simulink model "ModelSimulink"  (R2020a)
settings: Solver=VariableStepAuto  StartTime=0.0  StopTime=20  RelTol=1e-3
libraries: robotlib x50
settings Model: Creator=Ishmael  LastModifiedBy=Ishmael

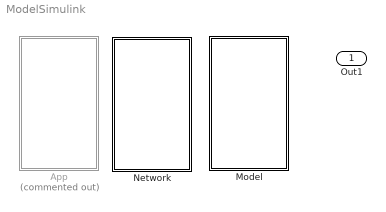
== system ModelSimulink ==
  App : Subsystem  Commented=on
  Model : Subsystem
  Network : Subsystem
  Out1 : Outport

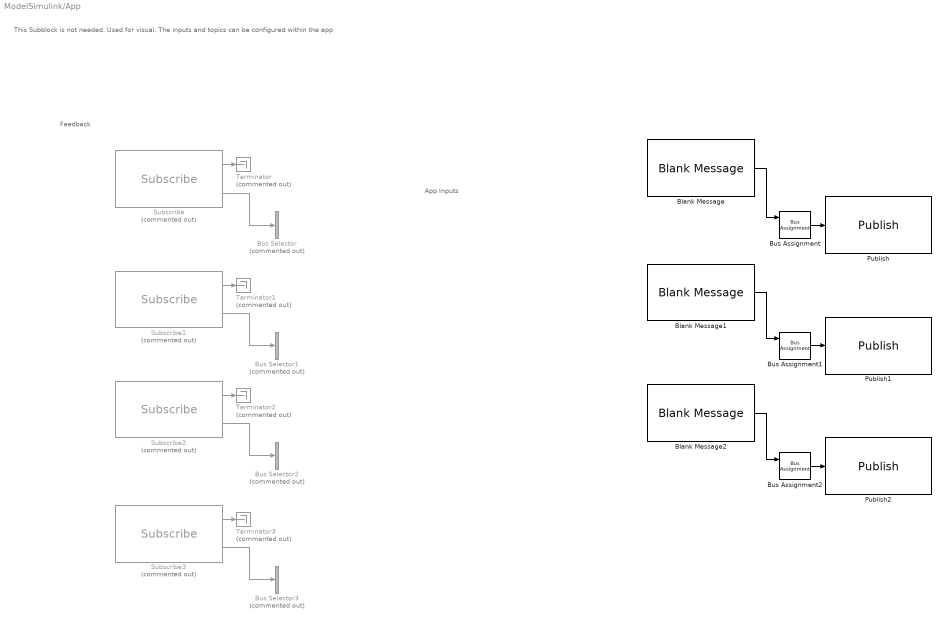
== system ModelSimulink/App ==
  note: This Subblock is not needed. Used for visual. The inputs and topics can be configured within the app
  note: App Inputs
  note: Feedback
  Blank Message : robotlib/Blank Message  messageClass=Message  entityType=geometry_msgs/Twist  messageType=geometry_msgs/Twist  SampleTime=inf
  Blank Message1 : robotlib/Blank Message  messageClass=Message  entityType=geometry_msgs/Twist  messageType=geometry_msgs/Twist  SampleTime=inf
  Blank Message2 : robotlib/Blank Message  messageClass=Message  entityType=geometry_msgs/Twist  messageType=geometry_msgs/Twist  SampleTime=inf
  Bus Assignment : BusAssignment  AssignedSignals=Linear.X
  Bus Assignment1 : BusAssignment  AssignedSignals=Linear.X
  Bus Assignment2 : BusAssignment  AssignedSignals=Linear.X
  Bus Selector{,1..3} (4 alike) : BusSelector  Commented=on  OutputSignals=Linear.X
  Publish : robotlib/Publish  topicSource=Select from ROS network  topic=/App/PedalPositionCommand  messageType=geometry_msgs/Twist  messageQueueLength=1
  Publish1 : robotlib/Publish  topicSource=Select from ROS network  topic=/App/SteeringPositionCommand  messageType=geometry_msgs/Twist  messageQueueLength=1
  Publish2 : robotlib/Publish  topicSource=Select from ROS network  topic=/App/SteeringPositionCommand  messageType=geometry_msgs/Twist  messageQueueLength=1
  Subscribe : robotlib/Subscribe  Commented=on  topicSource=Select from ROS network  topic=/App/CurrentPedalPosition  messageType=geometry_msgs/Twist  sampleTime=-1  messageQueueLength=1
  Subscribe1 : robotlib/Subscribe  Commented=on  topicSource=Select from ROS network  topic=/App/CurrentSteeringPosition  messageType=geometry_msgs/Twist  sampleTime=-1  messageQueueLength=1
  Subscribe2 : robotlib/Subscribe  Commented=on  topicSource=Select from ROS network  topic=/App/CurrentBreakingPosition  messageType=geometry_msgs/Twist  sampleTime=-1  messageQueueLength=1
  Subscribe3 : robotlib/Subscribe  Commented=on  topicSource=Select from ROS network  topic=/Model/Camera  messageType=geometry_msgs/Twist  sampleTime=-1  messageQueueLength=1
  Terminator{,1..3} (4 alike) : Terminator  Commented=on
  wires:
  Bus Assignment/1 -> Publish/1
  Blank Message/1 -> Bus Assignment/1
  ? -> Bus Assignment/2
  ? -> Bus Assignment1/2
  Blank Message1/1 -> Bus Assignment1/1
  Bus Assignment1/1 -> Publish1/1
  Bus Assignment2/1 -> Publish2/1
  Blank Message2/1 -> Bus Assignment2/1
  ? -> Bus Assignment2/2
  Subscribe/1 -> Terminator/1
  Subscribe/2 -> Bus Selector/1
  Subscribe1/2 -> Bus Selector1/1
  Subscribe1/1 -> Terminator1/1
  Subscribe2/1 -> Terminator2/1
  Subscribe2/2 -> Bus Selector2/1
  Subscribe3/2 -> Bus Selector3/1
  Subscribe3/1 -> Terminator3/1

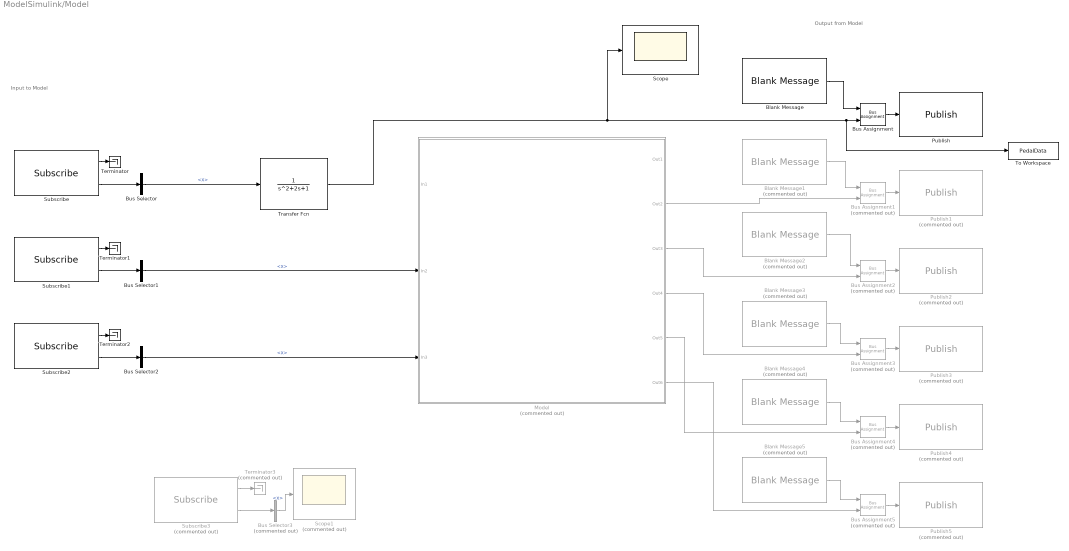
== system ModelSimulink/Model ==
  note: Input to Model
  note: Output from Model
  Blank Message : robotlib/Blank Message  messageClass=Message  entityType=geometry_msgs/Twist  messageType=geometry_msgs/Twist  SampleTime=inf
  Blank Message{1..5} (5 alike) : robotlib/Blank Message  Commented=on  messageClass=Message  entityType=geometry_msgs/Twist  messageType=geometry_msgs/Twist  SampleTime=inf
  Bus Assignment : BusAssignment  AssignedSignals=Linear.X
  Bus Assignment{1..5} (5 alike) : BusAssignment  Commented=on  AssignedSignals=Linear.X
  Bus Selector : BusSelector  OutputSignals=Linear.X
  Bus Selector1 : BusSelector  OutputSignals=Linear.X
  Bus Selector2 : BusSelector  OutputSignals=Linear.X
  Bus Selector3 : BusSelector  Commented=on  OutputSignals=Linear.X
  Model : Subsystem  Commented=on
  Publish : robotlib/Publish  topicSource=Select from ROS network  topic=/Model/PedalPositionReturn  messageType=geometry_msgs/Twist  messageQueueLength=1
  Publish1 : robotlib/Publish  Commented=on  topicSource=Select from ROS network  topic=/Model/SteeringPositionReturn  messageType=geometry_msgs/Twist  messageQueueLength=1
  Publish2 : robotlib/Publish  Commented=on  topicSource=Select from ROS network  topic=/Model/BreakingPositionReturn  messageType=geometry_msgs/Twist  messageQueueLength=1
  Publish3 : robotlib/Publish  Commented=on  topicSource=Select from ROS network  topic=/Model/Acceleration  messageType=geometry_msgs/Twist  messageQueueLength=1
  Publish4 : robotlib/Publish  Commented=on  topicSource=Select from ROS network  topic=/Model/TireAngle  messageType=geometry_msgs/Twist  messageQueueLength=1
  Publish5 : robotlib/Publish  Commented=on  topicSource=Select from ROS network  topic=/Model/Camera  messageType=geometry_msgs/Twist  messageQueueLength=1
  Scope : Scope
  Scope1 : Scope  Commented=on
  Subscribe : robotlib/Subscribe  topicSource=Select from ROS network  topic=/PedalPositionSend2m  messageType=geometry_msgs/Twist  sampleTime=-1  messageQueueLength=1
  Subscribe1 : robotlib/Subscribe  topicSource=Select from ROS network  topic=/SteeringPositionSend2m  messageType=geometry_msgs/Twist  sampleTime=-1  messageQueueLength=1
  Subscribe2 : robotlib/Subscribe  topicSource=Select from ROS network  topic=/BreakingPositionSend2m  messageType=geometry_msgs/Twist  sampleTime=-1  messageQueueLength=1
  Subscribe3 : robotlib/Subscribe  Commented=on  topicSource=Select from ROS network  topic=/Model/PedalPositionReturn  messageType=geometry_msgs/Twist  sampleTime=-1  messageQueueLength=1
  Terminator : Terminator
  Terminator1 : Terminator
  Terminator2 : Terminator
  Terminator3 : Terminator  Commented=on
  To Workspace : ToWorkspace  VariableName=PedalData  SaveFormat=Timeseries  SampleTime=-1
  Transfer Fcn : TransferFcn
  wires:
  Subscribe/1 -> Terminator/1
  Subscribe/2 -> Bus Selector/1
  Subscribe1/2 -> Bus Selector1/1
  Subscribe1/1 -> Terminator1/1
  Subscribe2/1 -> Terminator2/1
  Subscribe2/2 -> Bus Selector2/1
  Bus Selector2/1 -> Model/3(In3)  "<X>"
  Bus Selector/1 -> Transfer Fcn/1  "<X>"
  Bus Selector1/1 -> Model/2(In2)  "<X>"
  Bus Assignment/1 -> Publish/1
  Blank Message/1 -> Bus Assignment/1
  Model/2(Out2) -> Bus Assignment1/2
  Blank Message1/1 -> Bus Assignment1/1
  Bus Assignment1/1 -> Publish1/1
  Bus Assignment2/1 -> Publish2/1
  Blank Message2/1 -> Bus Assignment2/1
  Model/3(Out3) -> Bus Assignment2/2
  Model/4(Out4) -> Bus Assignment3/2
  Blank Message3/1 -> Bus Assignment3/1
  Bus Assignment3/1 -> Publish3/1
  Bus Assignment4/1 -> Publish4/1
  Blank Message4/1 -> Bus Assignment4/1
  Model/5(Out5) -> Bus Assignment4/2
  Model/6(Out6) -> Bus Assignment5/2
  Blank Message5/1 -> Bus Assignment5/1
  Bus Assignment5/1 -> Publish5/1
  Transfer Fcn/1 -> Scope/1, To Workspace/1, Bus Assignment/2
  Subscribe3/1 -> Terminator3/1
  Subscribe3/2 -> Bus Selector3/1
  Bus Selector3/1 -> Scope1/1  "<X>"

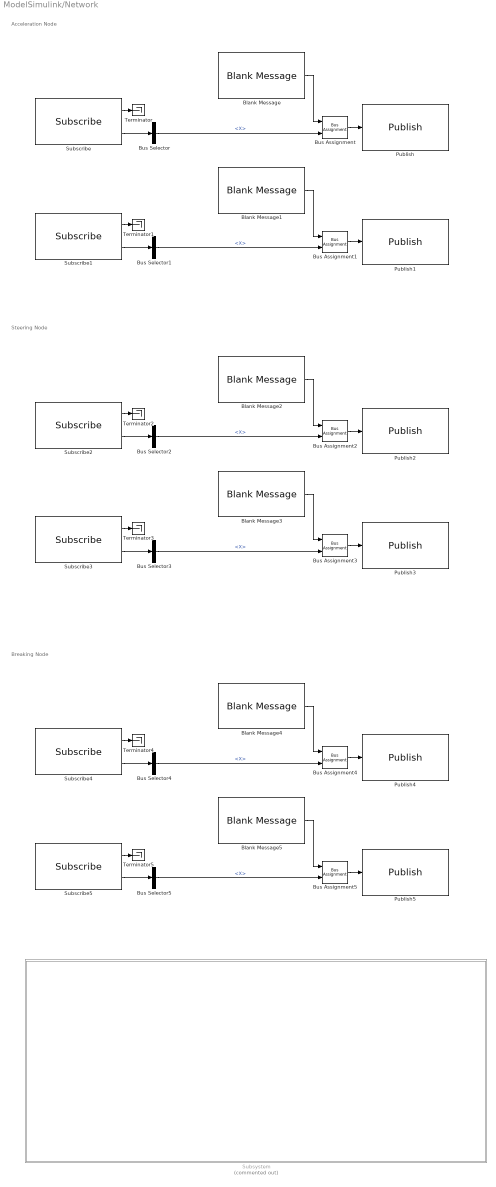
== system ModelSimulink/Network ==
  note: Acceleration Node
  note: Steering Node
  note: Breaking Node
  Blank Message{,1..5} (6 alike) : robotlib/Blank Message  messageClass=Message  entityType=geometry_msgs/Twist  messageType=geometry_msgs/Twist  SampleTime=inf
  Bus Assignment{,1..5} (6 alike) : BusAssignment  AssignedSignals=Linear.X
  Bus Selector{,1..5} (6 alike) : BusSelector  OutputSignals=Linear.X
  Publish : robotlib/Publish  topicSource=Select from ROS network  topic=/PedalPositionSend2m  messageType=geometry_msgs/Twist  messageQueueLength=1
  Publish1 : robotlib/Publish  topicSource=Select from ROS network  topic=/App/CurrentPedalPosition  messageType=geometry_msgs/Twist  messageQueueLength=1
  Publish2 : robotlib/Publish  topicSource=Select from ROS network  topic=/SteeringPositionSend2m  messageType=geometry_msgs/Twist  messageQueueLength=1
  Publish3 : robotlib/Publish  topicSource=Select from ROS network  topic=/App/CurrentSteeringPosition  messageType=geometry_msgs/Twist  messageQueueLength=1
  Publish4 : robotlib/Publish  topicSource=Select from ROS network  topic=/BreakingPositionSend2m  messageType=geometry_msgs/Twist  messageQueueLength=1
  Publish5 : robotlib/Publish  topicSource=Select from ROS network  topic=/App/CurrentBreakingPosition  messageType=geometry_msgs/Twist  messageQueueLength=1
  Subscribe : robotlib/Subscribe  topicSource=Select from ROS network  topic=/App/PedalPositionCommand  messageType=geometry_msgs/Twist  sampleTime=-1  messageQueueLength=1
  Subscribe1 : robotlib/Subscribe  topicSource=Select from ROS network  topic=/Model/PedalPositionReturn  messageType=geometry_msgs/Twist  sampleTime=-1  messageQueueLength=1
  Subscribe2 : robotlib/Subscribe  topicSource=Select from ROS network  topic=/App/SteeringPositionCommand  messageType=geometry_msgs/Twist  sampleTime=-1  messageQueueLength=1
  Subscribe3 : robotlib/Subscribe  topicSource=Select from ROS network  topic=/Model/SteeringPositionReturn  messageType=geometry_msgs/Twist  sampleTime=-1  messageQueueLength=1
  Subscribe4 : robotlib/Subscribe  topicSource=Select from ROS network  topic=/App/BreakingPositionCommand  messageType=geometry_msgs/Twist  sampleTime=-1  messageQueueLength=1
  Subscribe5 : robotlib/Subscribe  topicSource=Select from ROS network  topic=/Model/BreakingPositionReturn  messageType=geometry_msgs/Twist  sampleTime=-1  messageQueueLength=1
  Subsystem : Subsystem  Commented=on
  Terminator{,1..5} (6 alike) : Terminator
  wires:
  Blank Message/1 -> Bus Assignment/1
  Subscribe5/1 -> Terminator5/1
  Subscribe5/2 -> Bus Selector5/1
  Subscribe1/1 -> Terminator1/1
  Bus Assignment3/1 -> Publish3/1
  Blank Message5/1 -> Bus Assignment5/1
  Subscribe2/1 -> Terminator2/1
  Subscribe3/1 -> Terminator3/1
  Bus Assignment5/1 -> Publish5/1
  Bus Assignment1/1 -> Publish1/1
  Bus Selector5/1 -> Bus Assignment5/2  "<X>"
  Subscribe4/1 -> Terminator4/1
  Bus Selector2/1 -> Bus Assignment2/2  "<X>"
  Blank Message3/1 -> Bus Assignment3/1
  Bus Selector3/1 -> Bus Assignment3/2  "<X>"
  Bus Selector4/1 -> Bus Assignment4/2  "<X>"
  Subscribe1/2 -> Bus Selector1/1
  Blank Message2/1 -> Bus Assignment2/1
  Subscribe3/2 -> Bus Selector3/1
  Blank Message4/1 -> Bus Assignment4/1
  Subscribe2/2 -> Bus Selector2/1
  Subscribe/1 -> Terminator/1
  Bus Assignment2/1 -> Publish2/1
  Blank Message1/1 -> Bus Assignment1/1
  Bus Selector1/1 -> Bus Assignment1/2  "<X>"
  Bus Selector/1 -> Bus Assignment/2  "<X>"
  Subscribe/2 -> Bus Selector/1
  Bus Assignment/1 -> Publish/1
  Subscribe4/2 -> Bus Selector4/1
  Bus Assignment4/1 -> Publish4/1

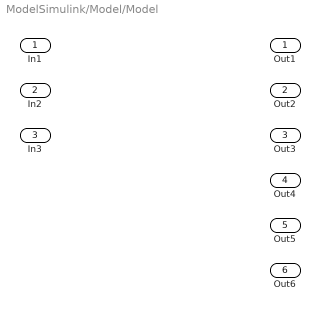
== system ModelSimulink/Model/Model ==
  In1 : Inport
  In2 : Inport  Port=2
  In3 : Inport  Port=3
  Out1 : Outport
  Out2 : Outport  Port=2
  Out3 : Outport  Port=3
  Out4 : Outport  Port=4
  Out5 : Outport  Port=5
  Out6 : Outport  Port=6

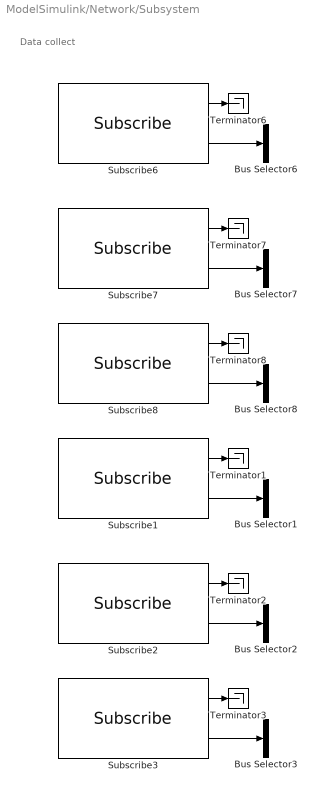
== system ModelSimulink/Network/Subsystem ==
  note: Data collect
  Bus Selector{1..3,6..8} (6 alike) : BusSelector  OutputSignals=Linear.X
  Subscribe1 : robotlib/Subscribe  topicSource=Select from ROS network  topic=/Model/Acceleration  messageType=geometry_msgs/Twist  sampleTime=-1  messageQueueLength=1
  Subscribe2 : robotlib/Subscribe  topicSource=Select from ROS network  topic=/Model/TireAngle  messageType=geometry_msgs/Twist  sampleTime=-1  messageQueueLength=1
  Subscribe3 : robotlib/Subscribe  topicSource=Select from ROS network  topic=/Model/Camera  messageType=geometry_msgs/Twist  sampleTime=-1  messageQueueLength=1
  Subscribe6 : robotlib/Subscribe  topicSource=Select from ROS network  topic=/Model/PedalPositionReturn  messageType=geometry_msgs/Twist  sampleTime=-1  messageQueueLength=1
  Subscribe7 : robotlib/Subscribe  topicSource=Select from ROS network  topic=/Model/SteeringPositionReturn  messageType=geometry_msgs/Twist  sampleTime=-1  messageQueueLength=1
  Subscribe8 : robotlib/Subscribe  topicSource=Select from ROS network  topic=/Model/BreakingPositionReturn  messageType=geometry_msgs/Twist  sampleTime=-1  messageQueueLength=1
  Terminator{1..3,6..8} (6 alike) : Terminator
  wires:
  Subscribe8/2 -> Bus Selector8/1
  Subscribe7/2 -> Bus Selector7/1
  Subscribe6/1 -> Terminator6/1
  Subscribe6/2 -> Bus Selector6/1
  Subscribe7/1 -> Terminator7/1
  Subscribe8/1 -> Terminator8/1
  Subscribe3/1 -> Terminator3/1
  Subscribe2/1 -> Terminator2/1
  Subscribe1/2 -> Bus Selector1/1
  Subscribe1/1 -> Terminator1/1
  Subscribe2/2 -> Bus Selector2/1
  Subscribe3/2 -> Bus Selector3/1
